simulink library "UserLibrary"  (Simulink 9.2)
settings: Solver=ode45  StartTime=0.0  StopTime=10.0  RelTol=1e-3  EnableMultiTasking=on
PostLoadFcn:
  | if any(exist('dsrtsu_mdlpostloadfcn', 'file') ~= 0), dsrtsu_mdlpostloadfcn('Execute', bdroot); end
undefined symbols (not defined in the file): ipReceive, ipSend, portReceive, portSend
libraries: slrealtimeiplib x2, xpclib x2, simulink x1
PreSaveFcn:
  | , if any(exist('dsmpb_private', 'file') ~= 0), dsmpb_private('dsmpb_mdlclblib', 'PreSave', bdroot); end,
CloseFcn:
  | , if any(exist('dsmpb_private', 'file') ~= 0), dsmpb_private('dsmpb_mdlclblib', 'Close', bdroot); end,
settings Model: DSMPB_ID_DATA={'110',struct('BlockId','3ebf5597-faf2-44bc-9be6-281b410fc813','SignalIds',{{'26d73f68-cffb-4ca0-bf58-82f7b62cb9ef','a5caa79d-886f-44a8-8d42-34ed95f43c78','1281cc26-2785-4f72-a4c1-cef9f3ba0f62','3fa82c26-d64d-4bba-bc5a-87026a128e33','9cb4c4fe-3056-46d2-91d7-6650514cac0e'}}),'123',struct('BlockId','5af8b6d2-464f-4b04-8812-8245578a7b3f','SignalIds',{{'8d80630f-4ba9-4581-af1d-b7a5605011a1'}})}  Creator=SeanK  LastModifiedBy=SeanKavanagh

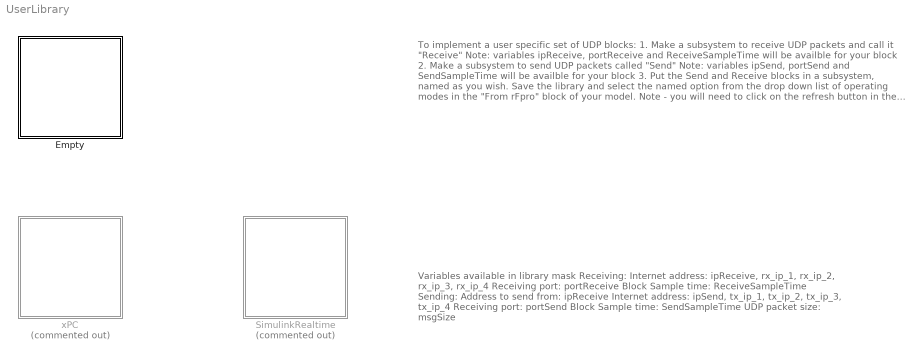
== system UserLibrary ==
  note: To implement a user specific set of UDP blocks:
      |
      | 1. Make a subsystem to receive UDP packets and call it "Receive"
      |         Note: variables ipReceive, portReceive and ReceiveSampleTime  will  be availble for your block
      | 2. Make a subsystem to send UDP packets called "Send"
      |         Note: variables ipSend, portSend and SendSampleTime  will  be availble for your block
      | 3. Put the Send and Receive blocks in a subsystem, named as you wish. Save the library and select the named option
      |     from the drop down list of operating modes in the "From rFpro" block of your model.
      |     Note - you will need to click on the refresh button in the mask once, and save the library to have the option
      |                available in future.
      |
      | Example blocks from various libraries are shown on the left.
      | Target specific blocks can be added using the Empty version as a starting point.
  note: Variables available in library mask
      |
      | Receiving:
      | Internet address: ipReceive, rx_ip_1, rx_ip_2, rx_ip_3, rx_ip_4
      | Receiving port: portReceive
      | Block Sample time: ReceiveSampleTime
      |
      | Sending:
      | Address to send from: ipReceive
      | Internet address: ipSend, tx_ip_1, tx_ip_2, tx_ip_3, tx_ip_4
      | Receiving port: portSend
      | Block Sample time: SendSampleTime
      | UDP packet size: msgSize
  Empty : Subsystem  Tag=struct('sysTarget', '', 'templateMakefile', '', 'makeCommand', '', 'description', 'Blank block for new hardware')
      settings: AttributesFormatString=|
      | Blank version - can be used as a
      | starting point for new UDP blocks
  SimulinkRealtime : Subsystem  Tag=struct('sysTarget', 'slrealtime.tlc', 'templateMakefile', '', 'makeCommand', '', 'description', '')  Commented=on
      settings: AttributesFormatString=|
      | Modern version of UDP blocks
      | from the Simulink realtime
      | library: slrealtimeiplib
  xPC : Subsystem  Tag=struct('sysTarget', 'xpctarget.tlc', 'templateMakefile', 'xpc_default_tmf', 'makeCommand', 'make_rtw', 'description', 'xPC target')  Commented=on
      settings: AttributesFormatString=|
      | Older version of UDP blocks
      | from the Simulink realtime
      | library: xpclib/UDP

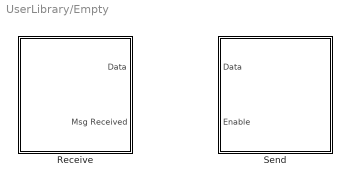
== system UserLibrary/Empty ==
  Receive : Subsystem
  Send : Subsystem

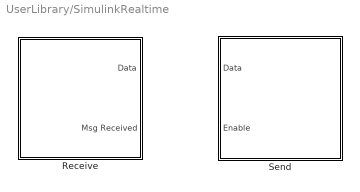
== system UserLibrary/SimulinkRealtime ==
  Receive : Subsystem  mask{ipVariable=ipReceive, portVariable=portReceive}
      mask prompts: ipVariable "Local IP Address"; portVariable "Local Port"
      mask init:
      | set_param([gcb '/Receive'], 'ipAddress', ipVariable);
      | set_param([gcb '/Receive'], 'localPort', num2str(portVariable));
  Send : Subsystem  mask{ipSourceVariable=ipReceive, ipTargetVariable=ipSend, portTargetVariable=portSend}
      mask prompts: ipSourceVariable "Local IP Address"; ipTargetVariable "Target IP Address"; portTargetVariable "Target Port"
      mask init:
      | set_param([gcb '/SendSubsystem/Send'], 'ipAddress', ipSourceVariable);
      | set_param([gcb '/SendSubsystem/Send'], 'toAddress', ipTargetVariable);
      | set_param([gcb '/SendSubsystem/Send'], 'toPort', num2str(portTargetVariable));

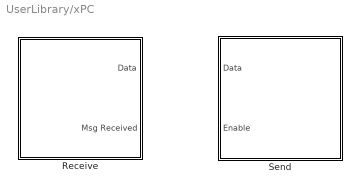
== system UserLibrary/xPC ==
  Receive : Subsystem  mask{ipVariable=ipReceive}
      mask prompts: ipVariable "Receiving address"
      mask init:
      | set_param([gcb '/Receive'], 'ipAddress', ipVariable)
  Send : Subsystem  mask{ipVariable=ipSend}
      mask prompts: ipVariable "IP Address to  Send To"
      mask init:
      | set_param([gcb '/xPC_Data_Send/Send'], 'ipAddress', ipVariable);

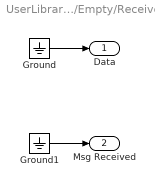
== system UserLibrary/Empty/Receive ==
  Ground : Ground
  Ground1 : Ground
  Data : Outport  OutDataTypeStr=uint8
  Msg Received : Outport  Port=2  OutDataTypeStr=boolean  PortDimensions=1
  wires:
  Ground/1 -> Data/1
  Ground1/1 -> Msg Received/1

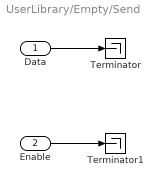
== system UserLibrary/Empty/Send ==
  Data : Inport  OutDataTypeStr=uint8
  Enable : Inport  Port=2  OutDataTypeStr=boolean  PortDimensions=1
  Terminator : Terminator
  Terminator1 : Terminator
  wires:
  Data/1 -> Terminator/1
  Enable/1 -> Terminator1/1

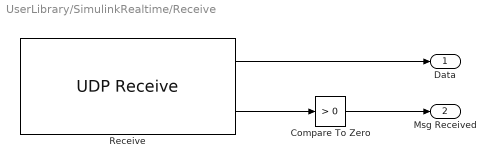
== system UserLibrary/SimulinkRealtime/Receive ==
  Compare To Zero : simulink/Logic and Bit Operations/Compare To Zero  relop=>  OutDataTypeStr=boolean
  Receive : slrealtimeiplib/UDP Receive  useHostTargetConn=off  ipAddress=127.0.0.1  localPort=11054  rcvWidth=2000  rcvFmAny=on  fmAddress=192.168.178.21  rcvMulticast=off  multicastAddress={}  sampleTime=ReceiveSampleTime
  Data : Outport
  Msg Received : Outport  Port=2
  wires:
  Receive/2 -> Compare To Zero/1
  Receive/1 -> Data/1
  Compare To Zero/1 -> Msg Received/1

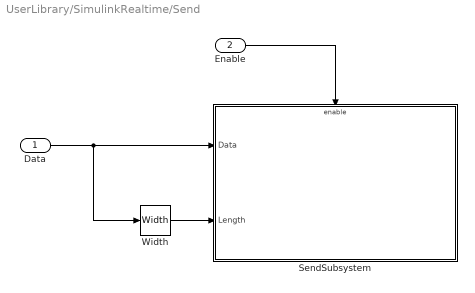
== system UserLibrary/SimulinkRealtime/Send ==
  Data : Inport
  Enable : Inport  Port=2
  SendSubsystem : Subsystem  TreatAsAtomicUnit=on
  Width : Width
  wires:
  Width/1 -> SendSubsystem/2(Length)
  Enable/1 -> SendSubsystem/Enable
  Data/1 -> Width/1, SendSubsystem/1(Data)

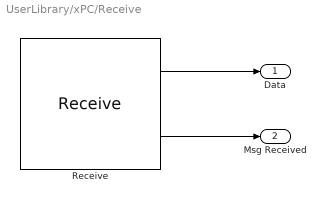
== system UserLibrary/xPC/Receive ==
  Receive : xpclib/UDP/Receive  ipAddress=127.0.0.1  ipPort=portReceive  width=2000  vblLen=on  sampletime=ReceiveSampleTime
      settings: SourceProductName=Simulink Real-Time  SourceProductBaseCode=XP
  Data : Outport
  Msg Received : Outport  Port=2
  wires:
  Receive/1 -> Data/1
  Receive/2 -> Msg Received/1

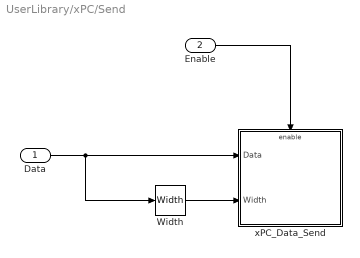
== system UserLibrary/xPC/Send ==
  Data : Inport
  Enable : Inport  Port=2
  Width : Width
  xPC_Data_Send : Subsystem  TreatAsAtomicUnit=on
  wires:
  Enable/1 -> xPC_Data_Send/Enable
  Data/1 -> Width/1, xPC_Data_Send/1(Data)
  Width/1 -> xPC_Data_Send/2(Width)

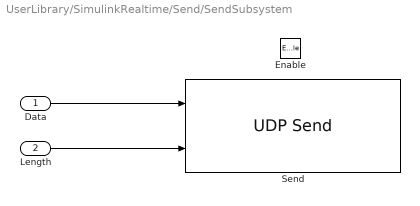
== system UserLibrary/SimulinkRealtime/Send/SendSubsystem ==
  Data : Inport
  Length : Inport  Port=2
  Enable : EnablePort
  Send : slrealtimeiplib/UDP Send  useHostTargetConn=off  ipAddress=127.0.0.1  localPort=-1  toAddress=127.0.0.1  toPort=11052  sampleTime=SendSampleTime
  wires:
  Data/1 -> Send/1
  Length/1 -> Send/2

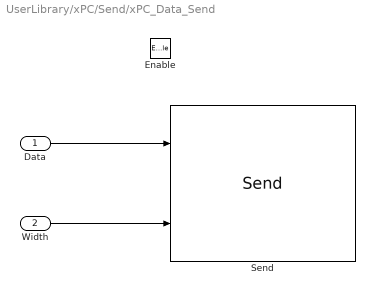
== system UserLibrary/xPC/Send/xPC_Data_Send ==
  Data : Inport
  Width : Inport  Port=2
  Enable : EnablePort
  Send : xpclib/UDP/Send  ipAddress=127.0.0.1  ipPort=portSend  localPort=-1  vblLen=on  sampletime=SendSampleTime
      settings: SourceProductName=Simulink Real-Time  SourceProductBaseCode=XP
  wires:
  Data/1 -> Send/1
  Width/1 -> Send/2
